simulink model "act2_espacio_de_estados"  (R2024a)
settings: Solver=VariableStepAuto  StartTime=0.0  StopTime=15  MaxStep=.001  RelTol=1e-3

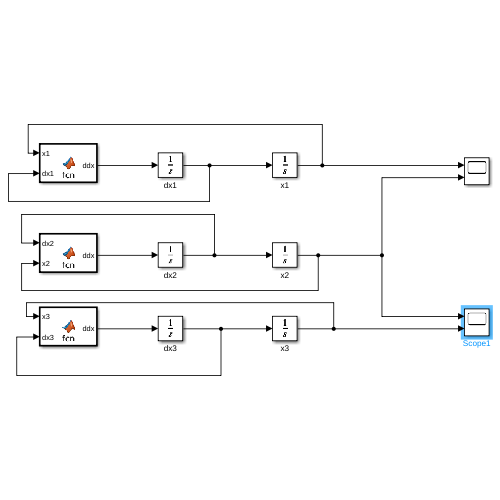
[thumbnail: Simulink's stored preview of the top-level diagram]
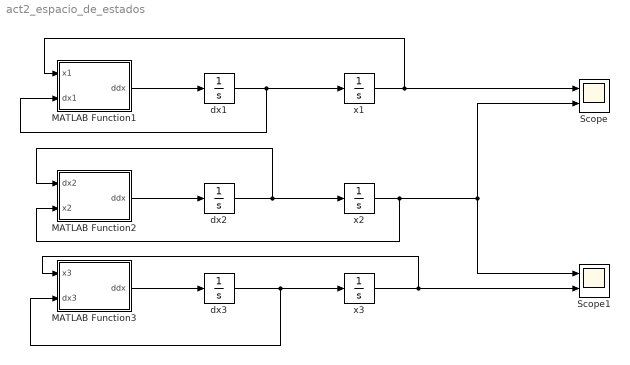
== system act2_espacio_de_estados ==
  MATLAB Function1 : MATLAB Function  TreatAsAtomicUnit=on
  MATLAB Function2 : MATLAB Function  TreatAsAtomicUnit=on
  MATLAB Function3 : MATLAB Function  TreatAsAtomicUnit=on
  Scope : Scope  NumInputPorts=2
  Scope1 : Scope  NumInputPorts=2
  dx1 : Integrator
  dx2 : Integrator
  dx3 : Integrator
  x1 : Integrator  InitialCondition=2*pi
  x2 : Integrator  InitialCondition=2*pi
  x3 : Integrator  InitialCondition=2*pi
  wires:
  MATLAB Function1/1(ddx) -> dx1/1
  dx1/1 -> MATLAB Function1/2(dx1), x1/1
  MATLAB Function2/1(ddx) -> dx2/1
  dx2/1 -> MATLAB Function2/1(dx2), x2/1
  x1/1 -> MATLAB Function1/1(x1), Scope/1
  x2/1 -> MATLAB Function2/2(x2), Scope1/1, Scope/2
  MATLAB Function3/1(ddx) -> dx3/1
  x3/1 -> MATLAB Function3/1(x3), Scope1/2
  dx3/1 -> MATLAB Function3/2(dx3), x3/1

== matlab function act2_espacio_de_estados/MATLAB Function3 ==
  data: x3 input; ddx output; dx3 input
function ddx = fcn(x3, dx3)
k = 0.01;
m = 0.75;
l = 0.36;
g = 9.8;
Tau = 0.5;
a = l/2;
J = .75 * m * (a*a);
ddx = (Tau/J) - ((k*dx3)/J) - ((m*g*a*x3)/J);

== matlab function act2_espacio_de_estados/MATLAB Function2 ==
  data: dx2 input; x2 input; ddx output
function ddx = fcn(dx2, x2)
k = 0.01;
m = 0.75;
l = 0.36;
g = 9.8;
Tau = 0.5;
a = l/2;
J = .75 * m * (a*a);
ddx = (Tau/J) - ((k*dx2)/J) - ((m*g*a*sin(x2))/J);

== matlab function act2_espacio_de_estados/MATLAB Function1 ==
  data: x1 input; dx1 input; ddx output
function ddx = fcn(x1, dx1)
k = 0.01;
m = 0.75;
l = 0.36;
g = 9.8;
Tau = 0.5;
a = l/2;
J = .75 * m * (a*a);
ddx = (Tau/J) - ((k*dx1)/J) - ((m*g*a*cos(x1))/J);
